simulink library "thc"  (R2021b)
settings: Solver=VariableStepAuto  StartTime=0.0  StopTime=10.0  RelTol=1e-3
undefined symbols (not defined in the file or in its folder): ATHC_APTCQA_X_C, ATHC_APTCQB_X_C, ATHC_dAy_X_C, ATHC_Qeq_X_kmh, ATHC_VbaseC_X_C, ATHC_VbaseC_Y_W, ATHC_VbaseD_X_C, ATHC_VbaseH_X_C, KTHC_ACMaxMinT_sec, KTHC_aDeice_K, KTHC_AGSDefLv_K, KTHC_AGSLv1_K, KTHC_AGSLv2_K, KTHC_AGSLv3_K, KTHC_AGSLv4_K, KTHC_AGSLv5_K, KTHC_AirIntUpdateT_sec, KTHC_APTCOneZoneMax_W, KTHC_APTCPeriod_cnt, KTHC_APTCPWMEN_flg, KTHC_APTCQMaxC_W, KTHC_APTCQminC_W, KTHC_APTCQminD_W, KTHC_APTCQminRe1_W, KTHC_APTCQminRe_W, KTHC_APTCQoffT_cnt, KTHC_APTCQonT_cnt, KTHC_APTCRiLeMaxDff_W, KTHC_APTCRiLeMinDff_W, KTHC_AutoWDTamb1_C, KTHC_AutoWDTamb2_C, KTHC_AutoWDTamb3_C, KTHC_BatCoolT_cnt, KTHC_BatInTempDef_C, KTHC_bDeice_K, KTHC_CompMaxDeice_rpm, KTHC_CompMinDeice_rpm, KTHC_CompSotxvOp_K, KTHC_CompSotxvOpLow_rpm, KTHC_CompSpdEXVUp1_rpm, KTHC_CompSpdEXVUp2_rpm, KTHC_CompSpdEXVUp3_rpm, KTHC_CompSpdEXVUp4_rpm, KTHC_CompSpdmax_rpm, KTHC_CompSpdmaxBC1_rpm, KTHC_CompSpdmaxBC_rpm, KTHC_CompSpdmid1_rpm, KTHC_CompSpdmid2_rpm, KTHC_CompSpdmid3_rpm, KTHC_CompSpdmid4_rpm, KTHC_CompSpdmid5_rpm, KTHC_CompSpdmid_rpm, KTHC_CompSpdmin_rpm, KTHC_DAPTCQ1_W, KTHC_DAPTCQ2_W, KTHC_DAPTCQ3_W, KTHC_DcChSetTemp_C, KTHC_DehumidityEN_flg, KTHC_DeiceCycTime_K, KTHC_DriveLevelWPTCBAH1_W ... (+403)
libraries: simulink x489
(part 2 of 18)

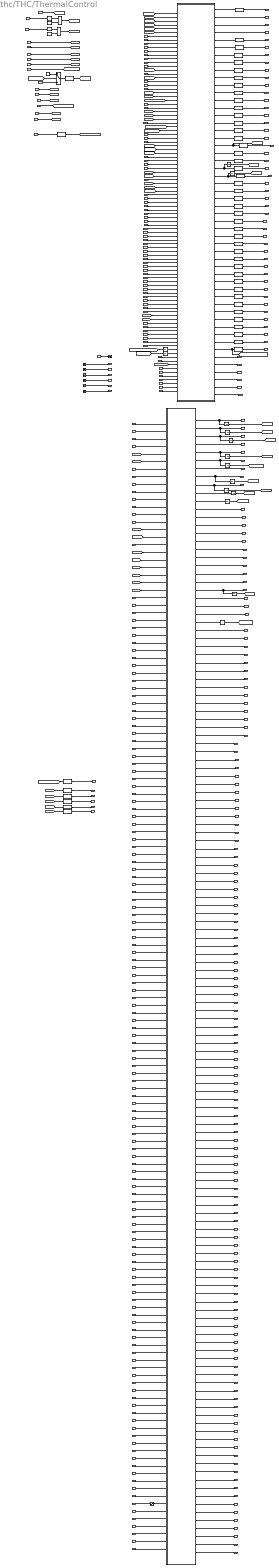
== system thc/THC/ThermalControl ==
  note: Ver Infomation
      | THCM Model V92A
      | ACHMI Model V33A
  VPMM_PwrSta_enum : Inport
  VPMM_SysPwrSta_enum : Inport  Port=2
  VTQD_ShiftGearPosn_enum : Inport  Port=3
  VSCP_AGSCloseSta_flg : Inport  Port=4
  VINP_VehSpeed_kph : Inport  Port=5
  VINP_HVBMTempMax_C : Inport  Port=6
  VINP_HVBMTempMin_C : Inport  Port=7
  VINP_OBCTemp_C : Inport  Port=8
  VINP_DCDCTemp_C : Inport  Port=9
  VINP_RrTMTemp_C : Inport  Port=10
  VINP_RrMCUTemp_C : Inport  Port=11
  VINP_FrTMTemp_C : Inport  Port=12
  VINP_FrMCUTemp_C : Inport  Port=13
  VINP_ChrgPlugSta_enum : Inport  Port=14
  VINP_FrLLCTemp_C : Inport  Port=15
  VINP_RrLLCTemp_C : Inport  Port=16
  VINP_HVBIsoImpedenceN_Mohm : Inport  Port=17
  VINP_HVBIsoImpedenceP_Mohm : Inport  Port=18
  VINP_HVBHVILErr_flg : Inport  Port=19
  VINP_HVBattSOC_pct : Inport  Port=20
  VINP_PTHighTact_C : Inport  Port=21
  VINP_COMP_StatorSpd_RPM : Inport  Port=22
  VINP_CompProEN_flg : Inport  Port=23
  VINP_PTLowP1_kPa : Inport  Port=24
  VINP_PTLowT1_C : Inport  Port=25
  VINP_PTLowP2_kPa : Inport  Port=26
  VINP_PTLowT2_C : Inport  Port=27
  VINP_PTHighP_kPa : Inport  Port=28
  VINP_Tamb_C : Inport  Port=29
  VINP_BatInTemp_C : Inport  Port=30
  VINP_BatOutTemp_C : Inport  Port=31
  VINP_MotorInTemp_C : Inport  Port=32
  VINP_MotorOutTemp_C : Inport  Port=33
  VINP_Tincar_C : Inport  Port=34
  VINP_SolarL_W : Inport  Port=35
  VINP_SolarR_W : Inport  Port=36
  VINP_Tevap_C : Inport  Port=37
  VINP_TFaceL_C : Inport  Port=38
  VINP_TFaceR_C : Inport  Port=39
  VINP_TFootL_C : Inport  Port=40
  VINP_TFootR_C : Inport  Port=41
  VINP_TFootRr_C : Inport  Port=42
  VINP_TFaceRr_C : Inport  Port=43
  VINP_EACProtectEnable_enum : Inport  Port=44
  Tamb_Err : Inport  Port=45
  SolarL_Err : Inport  Port=46
  SolarR_Err : Inport  Port=47
  Tevap_Err : Inport  Port=48
  T_Face_L_Err : Inport  Port=49
  T_Face_R_Err : Inport  Port=50
  T_Foot_L_Err : Inport  Port=51
  T_Foot_R_Err : Inport  Port=52
  T_Face_Rr_Err : Inport  Port=53
  T_Foot_Rr_Err : Inport  Port=54
  Tincar_Err : Inport  Port=55
  Bat_In_Temp_Err : Inport  Port=56
  Motor_In_Temp_Err : Inport  Port=57
  Motor_Out_Temp_Err : Inport  Port=58
  Fan_Err : Inport  Port=59
  AGS_Err : Inport  Port=60
  EWP3_Err : Inport  Port=61
  PT_High_P_Err : Inport  Port=62
  PT_High_Tact_Err : Inport  Port=63
  SOV1_Err : Inport  Port=64
  SOV2_Err : Inport  Port=65
  SOV3_Err : Inport  Port=66
  EXV1_Err : Inport  Port=67
  EXV2_Err : Inport  Port=68
  Comp_Err : Inport  Port=69
  Blower_Err : Inport  Port=70
  PT_Low_P1_Err : Inport  Port=71
  PT_Low_T1_Err : Inport  Port=72
  PT_Low_P2_Err : Inport  Port=73
  PT_Low_T2_Err : Inport  Port=74
  SOTXV_Err : Inport  Port=75
  VINP_FrntPTCRearLeActHeatPwr_W : Inport  Port=76
  VINP_FrntPTCLeActHeatPwr_W : Inport  Port=77
  VINP_FrntPTCRiActHeatPwr_W : Inport  Port=78
  VINP_ZFRTHCLEVentActYSta_enum : Inport  Port=79
  VINP_ZFRTHCCLEVentActYSta_enum : Inport  Port=80
  VINP_ZFRTHCREVentActYSta_enum : Inport  Port=81
  VINP_ZFRTHCCREVentActYSta_enum : Inport  Port=82
  VINP_FGSAirIntSta_enum : Inport  Port=83
  "VINP_EWP1BlockError_enum " : Inport  Port=84
  VINP_EWP1OverCurrError_enum : Inport  Port=85
  VINP_EWP2BlockError_enum : Inport  Port=86
  VINP_EWP2OverCurrError_enum : Inport  Port=87
  VINP_EWP3BlockError_enum : Inport  Port=88
  VINP_EWP3OverCurrError_enum : Inport  Port=89
  VINP_OFFACMODE_enum : Inport  Port=90
  VINP_FCPFrEvtBtnACMaxReq_flg : Inport  Port=91
  VINP_FCPFrEvtBtnACReq_flg : Inport  Port=92
  VINP_FCPFrEvtBtnAutoReq_flg : Inport  Port=93
  VINP_FCPFrEvtBtnSyncReq_flg : Inport  Port=94
  VINP_sigAirIntenZon1Req_enum : Inport  Port=95
  VINP_sigRecircReq_flg : Inport  Port=96
  VINP_sigFaceReq_flg : Inport  Port=97
  VINP_sigFootReq_flg : Inport  Port=98
  VINP_sigFrostReq_flg : Inport  Port=99
  VINP_sigSetTempZon1Req_C : Inport  Port=100
  VINP_CANMsgValidIVI2_flg : Inport  Port=101
  VINP_sigSetTempZon2Req_C : Inport  Port=102
  VINP_SmartEcoModeSW_flg : Inport  Port=103
  VINP_HMIACBtnCmd_flg : Inport  Port=104
  VINP_HMIACAutoBtnCmd_flg : Inport  Port=105
  VINP_HMIACRecycleBtnCmd_flg : Inport  Port=106
  VINP_HMIACFrDefogBtnCmd_flg : Inport  Port=107
  VINP_HMIZLSetTPCmd_flg : Inport  Port=108
  VINP_HMIZLSetTMCmd_flg : Inport  Port=109
  VINP_HMIZRSetTPCmd_flg : Inport  Port=110
  VINP_HMIZRSetTMCmd_flg : Inport  Port=111
  VINP_HMIACWindDirPCmd_flg : Inport  Port=112
  VINP_HMIACWindDirMCmd_flg : Inport  Port=113
  VINP_HMIACAirIntPCmd_flg : Inport  Port=114
  VINP_HMIACAirIntMCmd_flg : Inport  Port=115
  VINP_IVIAirIntZ3Cmd_enum : Inport  Port=116
  VINP_IVILBlowerModeSta_enum : Inport  Port=117
  VINP_IVIRBlowerModeSta_enum : Inport  Port=118
  VINP_IVILBlowerZSta_enum : Inport  Port=119
  VINP_IVICLBlowerZSta_enum : Inport  Port=120
  VINP_IVIRBlowerZSta_enum : Inport  Port=121
  VINP_IVICRBlowerZSta_enum : Inport  Port=122
  VINP_IVILBlowerYSta_enum : Inport  Port=123
  VINP_IVICLBlowerYSta_enum : Inport  Port=124
  VINP_IVIRBlowerYSta_enum : Inport  Port=125
  VINP_IVICRBlowerYSta_enum : Inport  Port=126
  VINP_IVIsigScreenReq_Sta : Inport  Port=127
  VINP_IVIFGSAirIntCmd_enum : Inport  Port=128
  VINP_IVIFGSChCmd_enum : Inport  Port=129
  VINP_IVIIONSWCmd_flg : Inport  Port=130
  VINP_IVIWPTCSWSta_flg : Inport  Port=131
  VINP_IVIZon1WindDirSWReqSta_flg : Inport  Port=132
  VINP_IVIQuickRefreshSta_flg : Inport  Port=133
  ECOSW : Inport  Port=134
  VINP_RemoteACTemp_C : Inport  Port=135
  VINP_RemoteAutoReq_flg : Inport  Port=136
  EEP_ACModeSet123 : Inport  Port=137
  EEP_FACESet : Inport  Port=138
  EEP_FOOTSet : Inport  Port=139
  EEP_FrostSet : Inport  Port=140
  EEP_FaceMSet : Inport  Port=141
  EEP_FootMSet : Inport  Port=142
  EEP_CCUSyncStsSet : Inport  Port=143
  EEP_sigRecircStSet : Inport  Port=144
  EEP_RecyAutoSet : Inport  Port=145
  EEP_AirIntenZone1MSet1 : Inport  Port=146
  EEP_fdefogSet : Inport  Port=147
  EEP_SettempZon1Set1 : Inport  Port=148
  EEP_sigSetTempZon2StM : Inport  Port=149
  EEP_AirIntenZone3MSet1 : Inport  Port=150
  EEP_FDCTHCREVentModeStaSet123 : Inport  Port=151
  EEP_FDCTHCLEVentModeStaSet123 : Inport  Port=152
  EEP_FDCTHCLEVentZStaSet1 : Inport  Port=153
  EEP_FDCTHCCLEVentZStaSet1 : Inport  Port=154
  EEP_FDCTHCREVentZStaSet1 : Inport  Port=155
  EEP_FDCTHCCREVentZStaSet1 : Inport  Port=156
  EEP_LVentENSet : Inport  Port=157
  EEP_FDCTHCLEVentYStaSet1 : Inport  Port=158
  EEP_CLVentENSet : Inport  Port=159
  EEP_FDCTHCCLEVentYStaSet1 : Inport  Port=160
  EEP_RVentENSet : Inport  Port=161
  EEP_FDCTHCREVentYStaSet1 : Inport  Port=162
  EEP_CRVentENSet : Inport  Port=163
  EEP_FDCTHCCREVentYStaSet1 : Inport  Port=164
  EEP_FDCFGSAirIntStaSet123 : Inport  Port=165
  EEP_FDCFGSChStaSet123 : Inport  Port=166
  EEP_IONSWStaSet : Inport  Port=167
  EEP_AirIntenZone1MSet2 : Inport  Port=168
  EEP_AirIntenZone1MSet3 : Inport  Port=169
  EEP_AirIntenZone1MSet4 : Inport  Port=170
  EEP_AirIntenZone1MSet5 : Inport  Port=171
  EEP_AirIntenZone1MSet7 : Inport  Port=172
  EEP_AirIntenZone3MSet2 : Inport  Port=173
  EEP_AirIntenZone3MSet3 : Inport  Port=174
  EEP_AirIntenZone3MSet4 : Inport  Port=175
  EEP_AirIntenZone3MSet5 : Inport  Port=176
  EEP_AirIntenZone3MSet7 : Inport  Port=177
  EEP_FDCFGSChStaSet457 : Inport  Port=178
  EEP_FDCFGSAirIntStaSet457 : Inport  Port=179
  EEP_FDCTHCLEVentModeStaSet457 : Inport  Port=180
  EEP_FDCTHCREVentModeStaSet457 : Inport  Port=181
  EEP_FDCTHCLEVentZStaSet2 : Inport  Port=182
  EEP_FDCTHCLEVentZStaSet3 : Inport  Port=183
  EEP_FDCTHCLEVentZStaSet4 : Inport  Port=184
  EEP_FDCTHCLEVentZStaSet5 : Inport  Port=185
  EEP_FDCTHCLEVentZStaSet7 : Inport  Port=186
  EEP_FDCTHCCLEVentZStaSet2 : Inport  Port=187
  EEP_FDCTHCCLEVentZStaSet3 : Inport  Port=188
  EEP_FDCTHCCLEVentZStaSet4 : Inport  Port=189
  EEP_FDCTHCCLEVentZStaSet5 : Inport  Port=190
  EEP_FDCTHCCLEVentZStaSet7 : Inport  Port=191
  EEP_FDCTHCREVentZStaSet2 : Inport  Port=192
  EEP_FDCTHCREVentZStaSet3 : Inport  Port=193
  EEP_FDCTHCREVentZStaSet4 : Inport  Port=194
  EEP_FDCTHCREVentZStaSet5 : Inport  Port=195
  EEP_FDCTHCREVentZStaSet7 : Inport  Port=196
  EEP_FDCTHCCREVentZStaSet2 : Inport  Port=197
  EEP_FDCTHCCREVentZStaSet3 : Inport  Port=198
  EEP_FDCTHCCREVentZStaSet4 : Inport  Port=199
  EEP_FDCTHCCREVentZStaSet5 : Inport  Port=200
  EEP_FDCTHCCREVentZStaSet7 : Inport  Port=201
  EEP_FDCTHCLEVentYStaSet2 : Inport  Port=202
  EEP_FDCTHCLEVentYStaSet3 : Inport  Port=203
  EEP_FDCTHCLEVentYStaSet4 : Inport  Port=204
  EEP_FDCTHCLEVentYStaSet5 : Inport  Port=205
  EEP_FDCTHCLEVentYStaSet7 : Inport  Port=206
  EEP_FDCTHCCLEVentYStaSet2 : Inport  Port=207
  EEP_FDCTHCCLEVentYStaSet3 : Inport  Port=208
  EEP_FDCTHCCLEVentYStaSet4 : Inport  Port=209
  EEP_FDCTHCCLEVentYStaSet5 : Inport  Port=210
  EEP_FDCTHCCLEVentYStaSet7 : Inport  Port=211
  EEP_FDCTHCREVentYStaSet2 : Inport  Port=212
  EEP_FDCTHCREVentYStaSet3 : Inport  Port=213
  EEP_FDCTHCREVentYStaSet4 : Inport  Port=214
  EEP_FDCTHCREVentYStaSet5 : Inport  Port=215
  EEP_FDCTHCREVentYStaSet7 : Inport  Port=216
  EEP_FDCTHCCREVentYStaSet2 : Inport  Port=217
  EEP_FDCTHCCREVentYStaSet3 : Inport  Port=218
  EEP_FDCTHCCREVentYStaSet4 : Inport  Port=219
  EEP_FDCTHCCREVentYStaSet5 : Inport  Port=220
  EEP_FDCTHCCREVentYStaSet7 : Inport  Port=221
  EEP_ACModeSet457 : Inport  Port=222
  EEP_SettempZon1Set2 : Inport  Port=223
  EEP_SettempZon1Set3 : Inport  Port=224
  EEP_SettempZon1Set4 : Inport  Port=225
  EEP_SettempZon1Set5 : Inport  Port=226
  EEP_SettempZon1Set7 : Inport  Port=227
  VBCM_UserNow_enum : Inport  Port=228
  VINP_UpdateReq_enum : Inport  Port=229
  APTCFailDTC : Inport  Port=230
  AC : Subsystem
  Abs : Abs
  Abs1 : Abs
  Constant : Constant
  Constant1 : Constant
  Constant2 : Constant  Value=2
  Data Type Conversion{,1..47,50} (49 alike) : DataTypeConversion
  Data Type Conversion48 : DataTypeConversion  OutDataTypeStr=uint8
  Data Type Conversion49 : DataTypeConversion  OutDataTypeStr=uint16
  Ground{,1..5} (6 alike) : Ground
  Max : MinMax  Function=max  Inputs=2
  Max1 : MinMax  Function=max  Inputs=2
  Saturation : Saturate  UpperLimit=30  LowerLimit=0
  Switch : Switch  Criteria=u2 > Threshold
  THCM_Conctrl : Subsystem
  Terminator : Terminator
  Unit Delay{,1..14} (15 alike) : UnitDelay  SampleTime=-1  HasFrameUpgradeWarning=on
  VTHC_FDCompCmd_rpm : Outport
  VTHC_FDSOV1Cmd_flg : Outport  Port=2
  VTHC_FDSOV2Cmd_flg : Outport  Port=3
  VTHC_FDSOV3Cmd_flg : Outport  Port=4
  VTHC_FDEXV1Cmd_step : Outport  Port=5
  VTHC_FDEXV2Cmd_step : Outport  Port=6
  VTHC_FDSOTXVCmd_flg : Outport  Port=7
  VTHC_FDFWVCmd_flg : Outport  Port=8
  VTHC_FDTWVCmd_pct : Outport  Port=9
  VTHC_FDFrWPTCHeatPwrCmd_W : Outport  Port=10
  VTHC_CoolgFanActDuty_pct : Outport  Port=11
  VTHC_FDAGSCmd_enum : Outport  Port=12
  VTHC_FDEWP1Cmd_enum : Outport  Port=13
  VTHC_FDEWP2Cmd_enum : Outport  Port=14
  VTHC_FDEWP3Cmd_enum : Outport  Port=15
  VTHC_FDFrLeAPTCHeatPwrCmd_W : Outport  Port=16
  VTHC_FDFrRiAPTCHeatPwrCmd_W : Outport  Port=17
  VTHC_FDRrAPTCHeatPwrCmd_W : Outport  Port=18
  VTHC_FDBlowerCmd_pct : Outport  Port=19
  VTHC_BatteryMode_enum : Outport  Port=20
  VTHC_EDriveMode_enum : Outport  Port=21
  VTHC_CabinMode_enum : Outport  Port=22
  VTHC_CCUACLampSts_flg : Outport  Port=23
  VTHC_CCUAutoLampSts_flg : Outport  Port=24
  VTHC_CCUACMaxLampSts_flg : Outport  Port=25
  VTHC_CCUSyncLampSts_flg : Outport  Port=26
  VTHC_sigAirIntenZon1St_enum : Outport  Port=27
  VTHC_sigWindDirZon1St_enum : Outport  Port=28
  VTHC_sigRecircSt_flg : Outport  Port=29
  VTHC_sigSetTempZon1St_C : Outport  Port=30
  VTHC_sigSetTempZon2St_C : Outport  Port=31
  VTHC_sigClntTHvBattOut_C : Outport  Port=32
  VTHC_sigCbnSolarLeft_W : Outport  Port=33
  VTHC_sigClntTHvBattIn_C : Outport  Port=34
  VTHC_sigCbnSolarRight_W : Outport  Port=35
  VTHC_sigAmbAirT_C : Outport  Port=36
  VTHC_sigCbnAirT_C : Outport  Port=37
  VTHC_ACSubMode_enum : Outport  Port=38
  VTHC_FDRecyAutoCmd_enum : Outport  Port=39
  VTHC_CompP_K : Outport  Port=40
  VTHC_CompI_K : Outport  Port=41
  VTHC_CompU_K : Outport  Port=42
  VTHC_CompDeltaU_K : Outport  Port=43
  VTHC_Compe_K : Outport  Port=44
  VTHC_Blowere_K : Outport  Port=45
  VTHC_BlowerP_K : Outport  Port=46
  VTHC_BlowerU_K : Outport  Port=47
  VTHC_Vbase_pct : Outport  Port=48
  VTHC_BlowerI_K : Outport  Port=49
  VTHC_EXV2P_K : Outport  Port=50
  VTHC_EXV2I_K : Outport  Port=51
  VTHC_EXV2U_K : Outport  Port=52
  VTHC_EXV2e_K : Outport  Port=53
  VTHC_APTCP_K : Outport  Port=54
  VTHC_APTCI_K : Outport  Port=55
  VTHC_APTCU_K : Outport  Port=56
  VTHC_APTCe_K : Outport  Port=57
  VTHC_EXV1P_K : Outport  Port=58
  VTHC_EXV1I_K : Outport  Port=59
  VTHC_EXV1U_K : Outport  Port=60
  VTHC_EXV1e_K : Outport  Port=61
  VTHC_ACModeMem_enum : Outport  Port=62
  VTHC_Face_flg : Outport  Port=63
  VTHC_Foot_flg : Outport  Port=64
  VTHC_Frost_flg : Outport  Port=65
  VTHC_FaceM_flg : Outport  Port=66
  VTHC_FootM_flg : Outport  Port=67
  VTHC_CCUSyncSts_flg : Outport  Port=68
  VTHC_RecAutoFlg_flg : Outport  Port=69
  VTHC_AirIntenZone1M_enum : Outport  Port=70
  VTHC_fdefog_flg : Outport  Port=71
  VTHC_sigSetTempZon2StM_C : Outport  Port=72
  VTHC_sigDfrstSt_flg : Outport  Port=73
  VTHC_FDCTHCAirIntZ3Sta_enum : Outport  Port=74
  VTHC_FDCTHCLEVentModeSta_enum : Outport  Port=75
  VTHC_FDCTHCREVentModeSta_enum : Outport  Port=76
  VTHC_FDCTHCLEVentZSta_enum : Outport  Port=77
  VTHC_FDCTHCCLEVentZSta_enum : Outport  Port=78
  VTHC_FDCTHCREVentZSta_enum : Outport  Port=79
  VTHC_FDCTHCCREVentZSta_enum : Outport  Port=80
  VTHC_FDCTHCLEVentYSta_enum : Outport  Port=81
  VTHC_FDCTHCLVentENSta_flg : Outport  Port=82
  VTHC_FDCTHCCLEVentYSta_enum : Outport  Port=83
  VTHC_FDCTHCCLVentENSta_flg : Outport  Port=84
  VTHC_FDCTHCREVentYSta_enum : Outport  Port=85
  VTHC_FDCTHCRVentENSta_flg : Outport  Port=86
  VTHC_FDCTHCCREVentYSta_enum : Outport  Port=87
  VTHC_FDCTHCCRVentENSta_flg : Outport  Port=88
  VTHC_FDCTHCMAPTCForceOFFSta_flg : Outport  Port=89
  VTHC_Z1TUP_flg : Outport  Port=90
  VTHC_Z1TDN_flg : Outport  Port=91
  VTHC_Z2TUP_flg : Outport  Port=92
  VTHC_Z2TDN_flg : Outport  Port=93
  VTHC_FDCFGSAirIntSta_enum : Outport  Port=94
  VTHC_FDCFGSChSta_enum : Outport  Port=95
  VTHC_FDCFGSAirIntCmd_enum : Outport  Port=96
  VTHC_FDCFGSFuncSta_enum : Outport  Port=97
  VTHC_FDCFGSChCmd_enum : Outport  Port=98
  VTHC_FDCFGSIONSWSta_flg : Outport  Port=99
  VTHC_FDCFGSIONCmd_flg : Outport  Port=100
  VTHC_FDCTHCMPreWPTCHeatSta_enum : Outport  Port=101
  VTHC_EWPBUflag1_flg : Outport  Port=102
  VTHC_EWPBUflag2_flg : Outport  Port=103
  VTHC_EWPBUflag3_flg : Outport  Port=104
  VTHC_FaceMSet_enum : Outport  Port=105
  VTHC_FootMSet_enum : Outport  Port=106
  VTHC_fdefogSet_enum : Outport  Port=107
  VTHC_CCUSyncStsSet_enum : Outport  Port=108
  VTHC_sigRecircStSet_enum : Outport  Port=109
  VTHC_RecyAutoSet_enum : Outport  Port=110
  VTHC_AirIntenZone1MSet1_enum : Outport  Port=111
  VTHC_AirIntenZone1MSet2_enum : Outport  Port=112
  VTHC_AirIntenZone1MSet3_enum : Outport  Port=113
  VTHC_AirIntenZone1MSet4_enum : Outport  Port=114
  VTHC_AirIntenZone1MSet5_enum : Outport  Port=115
  VTHC_AirIntenZone1MSet7_enum : Outport  Port=116
  VTHC_AirIntenZone3MSet1_enum : Outport  Port=117
  VTHC_AirIntenZone3MSet2_enum : Outport  Port=118
  VTHC_AirIntenZone3MSet3_enum : Outport  Port=119
  VTHC_AirIntenZone3MSet4_enum : Outport  Port=120
  VTHC_AirIntenZone3MSet5_enum : Outport  Port=121
  VTHC_AirIntenZone3MSet7_enum : Outport  Port=122
  VTHC_IONSWStaSet_enum : Outport  Port=123
  VTHC_FDCFGSChStaSet123_enum : Outport  Port=124
  VTHC_FDCFGSChStaSet457_enum : Outport  Port=125
  VTHC_FDCFGSAirIntStaSet123_enum : Outport  Port=126
  VTHC_FDCFGSAirIntStaSet457_enum : Outport  Port=127
  VTHC_LVentENSet_enum : Outport  Port=128
  VTHC_CLVentENSet_enum : Outport  Port=129
  VTHC_RVentENSet_enum : Outport  Port=130
  VTHC_CRVentENSet_enum : Outport  Port=131
  VTHC_LEVentModeStaSet123_enum : Outport  Port=132
  VTHC_LEVentModeStaSet457_enum : Outport  Port=133
  VTHC_REVentModeStaSet123_enum : Outport  Port=134
  VTHC_REVentModeStaSet457_enum : Outport  Port=135
  VTHC_FDCTHCLEVentZStaSet1_enum : Outport  Port=136
  VTHC_FDCTHCLEVentZStaSet2_enum : Outport  Port=137
  VTHC_FDCTHCLEVentZStaSet3_enum : Outport  Port=138
  VTHC_FDCTHCLEVentZStaSet4_enum : Outport  Port=139
  VTHC_FDCTHCLEVentZStaSet5_enum : Outport  Port=140
  VTHC_FDCTHCLEVentZStaSet7_enum : Outport  Port=141
  VTHC_FDCTHCCLEVentZStaSet1_enum : Outport  Port=142
  VTHC_FDCTHCCLEVentZStaSet2_enum : Outport  Port=143
  VTHC_FDCTHCCLEVentZStaSet3_enum : Outport  Port=144
  VTHC_FDCTHCCLEVentZStaSet4_enum : Outport  Port=145
  VTHC_FDCTHCCLEVentZStaSet5_enum : Outport  Port=146
  VTHC_FDCTHCCLEVentZStaSet7_enum : Outport  Port=147
  VTHC_FDCTHCREVentZStaSet1_enum : Outport  Port=148
  VTHC_FDCTHCREVentZStaSet2_enum : Outport  Port=149
  VTHC_FDCTHCREVentZStaSet3_enum : Outport  Port=150
  VTHC_FDCTHCREVentZStaSet4_enum : Outport  Port=151
  VTHC_FDCTHCREVentZStaSet5_enum : Outport  Port=152
  VTHC_FDCTHCREVentZStaSet7_enum : Outport  Port=153
  VTHC_FDCTHCCREVentZStaSet1_enum : Outport  Port=154
  VTHC_FDCTHCCREVentZStaSet2_enum : Outport  Port=155
  VTHC_FDCTHCCREVentZStaSet3_enum : Outport  Port=156
  VTHC_FDCTHCCREVentZStaSet4_enum : Outport  Port=157
  VTHC_FDCTHCCREVentZStaSet5_enum : Outport  Port=158
  VTHC_FDCTHCCREVentZStaSet7_enum : Outport  Port=159
  VTHC_FDCTHCLEVentYStaSet1_enum : Outport  Port=160
  VTHC_FDCTHCLEVentYStaSet2_enum : Outport  Port=161
  VTHC_FDCTHCLEVentYStaSet3_enum : Outport  Port=162
  VTHC_FDCTHCLEVentYStaSet4_enum : Outport  Port=163
  VTHC_FDCTHCLEVentYStaSet5_enum : Outport  Port=164
  VTHC_FDCTHCLEVentYStaSet7_enum : Outport  Port=165
  VTHC_FDCTHCCLEVentYStaSet1_enum : Outport  Port=166
  VTHC_FDCTHCCLEVentYStaSet2_enum : Outport  Port=167
  VTHC_FDCTHCCLEVentYStaSet3_enum : Outport  Port=168
  VTHC_FDCTHCCLEVentYStaSet4_enum : Outport  Port=169
  VTHC_FDCTHCCLEVentYStaSet5_enum : Outport  Port=170
  VTHC_FDCTHCCLEVentYStaSet7_enum : Outport  Port=171
  VTHC_FDCTHCREVentYStaSet1_enum : Outport  Port=172
  VTHC_FDCTHCREVentYStaSet2_enum : Outport  Port=173
  VTHC_FDCTHCREVentYStaSet3_enum : Outport  Port=174
  VTHC_FDCTHCREVentYStaSet4_enum : Outport  Port=175
  VTHC_FDCTHCREVentYStaSet5_enum : Outport  Port=176
  VTHC_FDCTHCREVentYStaSet7_enum : Outport  Port=177
  VTHC_FDCTHCCREVentYStaSet1_enum : Outport  Port=178
  VTHC_FDCTHCCREVentYStaSet2_enum : Outport  Port=179
  VTHC_FDCTHCCREVentYStaSet3_enum : Outport  Port=180
  VTHC_FDCTHCCREVentYStaSet4_enum : Outport  Port=181
  VTHC_FDCTHCCREVentYStaSet5_enum : Outport  Port=182
  VTHC_FDCTHCCREVentYStaSet7_enum : Outport  Port=183
  VTHC_SettempZon1Set1_enum : Outport  Port=184
  VTHC_SettempZon1Set2_enum : Outport  Port=185
  VTHC_SettempZon1Set3_enum : Outport  Port=186
  VTHC_SettempZon1Set4_enum : Outport  Port=187
  VTHC_SettempZon1Set5_enum : Outport  Port=188
  VTHC_SettempZon1Set7_enum : Outport  Port=189
  VTHC_ACModeSet123_enum : Outport  Port=190
  VTHC_ACModeSet457_enum : Outport  Port=191
  VTHC_FACESet_enum : Outport  Port=192
  VTHC_FOOTSet_enum : Outport  Port=193
  VTHC_FrostSet_enum : Outport  Port=194
  VTHC_LVentEN_flg : Outport  Port=195
  VTHC_CLVentEN_flg : Outport  Port=196
  VTHC_RVentEN_flg : Outport  Port=197
  VTHC_CRVentEN_flg : Outport  Port=198
  VTHC_FDCFGSLearnCmd_enum : Outport  Port=199
  VTHC_FDCFGSFuncSta_flg : Outport  Port=200
  VTHC_THSysErrlampReq_flg : Outport  Port=201
  VTHC_sigCbnPTCPwrAct_W : Outport  Port=202
  wires:
  THCM_Conctrl/51(VTHC_THSysErrlampReq_flg) -> VTHC_THSysErrlampReq_flg/1  "VTHC_THSysErrlampReq_flg"
  VPMM_SysPwrSta_enum/1 -> THCM_Conctrl/101(VPMM_SysPwrSta_enum)
  Ground5/1 -> VTHC_FDCFGSFuncSta_flg/1  "VTHC_FDCFGSFuncSta_flg"
  Saturation/1 -> AC/144(EEP_SettempZon1Set1)
  Ground4/1 -> VTHC_FDCFGSLearnCmd_enum/1  "VTHC_FDCFGSLearnCmd_enum"
  Ground2/1 -> VTHC_RVentEN_flg/1  "VTHC_RVentEN_flg"
  Ground3/1 -> VTHC_CRVentEN_flg/1  "VTHC_CRVentEN_flg"
  Ground1/1 -> VTHC_CLVentEN_flg/1  "VTHC_CLVentEN_flg"
  Ground/1 -> VTHC_LVentEN_flg/1  "VTHC_LVentEN_flg"
  AC/56(FrostSet) -> VTHC_FrostSet_enum/1  "VTHC_FrostSet_enum"
  AC/55(FOOTSet) -> VTHC_FOOTSet_enum/1  "VTHC_FOOTSet_enum"
  AC/54(FACESet) -> VTHC_FACESet_enum/1  "VTHC_FACESet_enum"
  AC/53(ACModeSet457) -> VTHC_ACModeSet457_enum/1  "VTHC_ACModeSet457_enum"
  AC/52(ACModeSet123) -> VTHC_ACModeSet123_enum/1  "VTHC_ACModeSet123_enum"
  AC/51(VTHC_FDCFGSIONCmd_flg) -> VTHC_FDCFGSIONCmd_flg/1  "VTHC_FDCFGSIONCmd_flg"
  AC/50(VTHC_FDCFGSIONSWSta_flg) -> VTHC_FDCFGSIONSWSta_flg/1  "VTHC_FDCFGSIONSWSta_flg"
  AC/49(VTHC_FDCFGSChCmd_enum) -> VTHC_FDCFGSChCmd_enum/1  "VTHC_FDCFGSChCmd_enum"
  AC/48(VTHC_FDCFGSFuncSta_enum) -> VTHC_FDCFGSFuncSta_enum/1  "VTHC_FDCFGSFuncSta_enum"
  AC/47(VTHC_FDCFGSAirIntCmd_enum) -> VTHC_FDCFGSAirIntCmd_enum/1  "VTHC_FDCFGSAirIntCmd_enum"
  AC/46(VTHC_FDCFGSChSta_enum) -> VTHC_FDCFGSChSta_enum/1  "VTHC_FDCFGSChSta_enum"
  AC/45(VTHC_FDCFGSAirIntSta_enum) -> VTHC_FDCFGSAirIntSta_enum/1  "VTHC_FDCFGSAirIntSta_enum"
  AC/44(VTHC_Z2TDN_flg) -> VTHC_Z2TDN_flg/1  "VTHC_Z2TDN_flg"
  AC/43(VTHC_Z2TUP_flg) -> VTHC_Z2TUP_flg/1  "VTHC_Z2TUP_flg"
  AC/42(VTHC_Z1TDN_flg) -> VTHC_Z1TDN_flg/1  "VTHC_Z1TDN_flg"
  AC/41(VTHC_Z1TUP_flg) -> VTHC_Z1TUP_flg/1  "VTHC_Z1TUP_flg"
  EEP_SettempZon1Set7/1 -> AC/149(EEP_SettempZon1Set7)
  EEP_SettempZon1Set5/1 -> AC/148(EEP_SettempZon1Set5)
  EEP_SettempZon1Set4/1 -> AC/147(EEP_SettempZon1Set4)
  EEP_SettempZon1Set3/1 -> AC/146(EEP_SettempZon1Set3)
  EEP_SettempZon1Set2/1 -> AC/145(EEP_SettempZon1Set2)
  EEP_SettempZon1Set1/1 -> Saturation/1
  EEP_FDCTHCCREVentYStaSet7/1 -> AC/143(EEP_FDCTHCCREVentYStaSet7)
  EEP_FDCTHCCREVentYStaSet5/1 -> AC/142(EEP_FDCTHCCREVentYStaSet5)
  EEP_FDCTHCCREVentYStaSet4/1 -> AC/141(EEP_FDCTHCCREVentYStaSet4)
  EEP_FDCTHCCREVentYStaSet3/1 -> AC/140(EEP_FDCTHCCREVentYStaSet3)
  EEP_FDCTHCCREVentYStaSet2/1 -> AC/139(EEP_FDCTHCCREVentYStaSet2)
  EEP_FDCTHCCREVentYStaSet1/1 -> AC/138(EEP_FDCTHCCREVentYStaSet1)
  EEP_FDCTHCREVentYStaSet7/1 -> AC/137(EEP_FDCTHCREventYStaSet7)
  EEP_FDCTHCREVentYStaSet5/1 -> AC/136(EEP_FDCTHCREventYStaSet5)
  EEP_FDCTHCREVentYStaSet4/1 -> AC/135(EEP_FDCTHCREventYStaSet4)
  EEP_FDCTHCREVentYStaSet3/1 -> AC/134(EEP_FDCTHCREventYStaSet3)
  EEP_FDCTHCREVentYStaSet2/1 -> AC/133(EEP_FDCTHCREventYStaSet2)
  EEP_FDCTHCREVentYStaSet1/1 -> AC/132(EEP_FDCTHCREventYStaSet1)
  EEP_FDCTHCCLEVentYStaSet7/1 -> AC/131(EEP_FDCTHCCLEVentYStaSet7)
  EEP_FDCTHCCLEVentYStaSet5/1 -> AC/130(EEP_FDCTHCCLEVentYStaSet5)
  EEP_FDCTHCCLEVentYStaSet4/1 -> AC/129(EEP_FDCTHCCLEVentYStaSet4)
  EEP_FDCTHCCLEVentYStaSet3/1 -> AC/128(EEP_FDCTHCCLEVentYStaSet3)
  EEP_FDCTHCCLEVentYStaSet2/1 -> AC/127(EEP_FDCTHCCLEVentYStaSet2)
  EEP_FDCTHCCLEVentYStaSet1/1 -> AC/126(EEP_FDCTHCCLEVentYStaSet1)
  EEP_FDCTHCLEVentYStaSet7/1 -> AC/125(EEP_FDCTHCLEventYStaSet7)
  EEP_FDCTHCLEVentYStaSet5/1 -> AC/124(EEP_FDCTHCLEventYStaSet5)
  EEP_FDCTHCLEVentYStaSet4/1 -> AC/123(EEP_FDCTHCLEventYStaSet4)
  EEP_FDCTHCLEVentYStaSet3/1 -> AC/122(EEP_FDCTHCLEventYStaSet3)
  EEP_FDCTHCLEVentYStaSet2/1 -> AC/121(EEP_FDCTHCLEventYStaSet2)
  EEP_FDCTHCCREVentZStaSet7/1 -> AC/119(EEP_FDCTHCCREVentZStaSet7)
  EEP_FDCTHCLEVentYStaSet1/1 -> AC/120(EEP_FDCTHCLEventYStaSet1)
  EEP_FDCTHCCREVentZStaSet5/1 -> AC/118(EEP_FDCTHCCREVentZStaSet5)
  EEP_FDCTHCCREVentZStaSet4/1 -> AC/117(EEP_FDCTHCCREVentZStaSet4)
  EEP_FDCTHCCREVentZStaSet3/1 -> AC/116(EEP_FDCTHCCREVentZStaSet3)
  EEP_FDCTHCCREVentZStaSet2/1 -> AC/115(EEP_FDCTHCCREVentZStaSet2)
  EEP_FDCTHCCREVentZStaSet1/1 -> AC/114(EEP_FDCTHCCREVentZStaSet1)
  EEP_FDCTHCREVentZStaSet7/1 -> AC/113(EEP_FDCTHCREventZStaSet7)
  EEP_FDCTHCREVentZStaSet5/1 -> AC/112(EEP_FDCTHCREventZStaSet5)
  EEP_FDCTHCREVentZStaSet4/1 -> AC/111(EEP_FDCTHCREventZStaSet4)
  EEP_FDCTHCREVentZStaSet3/1 -> AC/110(EEP_FDCTHCREventZStaSet3)
  EEP_FDCTHCREVentZStaSet2/1 -> AC/109(EEP_FDCTHCREventZStaSet2)
  EEP_FDCTHCREVentZStaSet1/1 -> AC/108(EEP_FDCTHCREventZStaSet1)
  EEP_FDCTHCCLEVentZStaSet7/1 -> AC/107(EEP_FDCTHCCLEVentZStaSet7)
  EEP_FDCTHCCLEVentZStaSet5/1 -> AC/106(EEP_FDCTHCCLEVentZStaSet5)
  EEP_FDCTHCCLEVentZStaSet4/1 -> AC/105(EEP_FDCTHCCLEVentZStaSet4)
  EEP_FDCTHCCLEVentZStaSet3/1 -> AC/104(EEP_FDCTHCCLEVentZStaSet3)
  EEP_FDCTHCCLEVentZStaSet2/1 -> AC/103(EEP_FDCTHCCLEVentZStaSet2)
  EEP_FDCTHCCLEVentZStaSet1/1 -> AC/102(EEP_FDCTHCCLEVentZStaSet1)
  EEP_FDCTHCLEVentZStaSet7/1 -> AC/101(EEP_FDCTHCLEventZStaSet7)
  EEP_FDCTHCLEVentZStaSet5/1 -> AC/100(EEP_FDCTHCLEventZStaSet5)
  EEP_FDCTHCLEVentZStaSet4/1 -> AC/99(EEP_FDCTHCLEventZStaSet4)
  EEP_FDCTHCLEVentZStaSet3/1 -> AC/98(EEP_FDCTHCLEventZStaSet3)
  EEP_FDCTHCLEVentZStaSet2/1 -> AC/97(EEP_FDCTHCLEventZStaSet2)
  EEP_FDCTHCLEVentZStaSet1/1 -> AC/96(EEP_FDCTHCLEventZStaSet1)
  EEP_FDCTHCREVentModeStaSet457/1 -> AC/95(EEP_FDCTHCREventModeStaSet457)
  EEP_FDCTHCREVentModeStaSet123/1 -> AC/94(EEP_FDCTHCREventModeStaSet123)
  EEP_FDCTHCLEVentModeStaSet457/1 -> AC/93(EEP_FDCTHCLEventModeStaSet457)
  EEP_FDCTHCLEVentModeStaSet123/1 -> AC/92(EEP_FDCTHCLEventModeStaSet123)
  EEP_CRVentENSet/1 -> AC/91(EEP_CRVentENSet)
  EEP_RVentENSet/1 -> AC/90(EEP_RVentENSet)
  EEP_CLVentENSet/1 -> AC/89(EEP_CLVentENSet)
  EEP_LVentENSet/1 -> AC/88(EEP_LVentENSet)
  EEP_FDCFGSAirIntStaSet457/1 -> AC/87(EEP_FDCFGSAirIntStaSet457)
  EEP_FDCFGSAirIntStaSet123/1 -> AC/86(EEP_FDCFGSAirIntStaSet123)
  EEP_FDCFGSChStaSet457/1 -> AC/85(EEP_FDCFGSChStaSet457)
  EEP_FDCFGSChStaSet123/1 -> AC/84(EEP_FDCFGSChStaSet123)
  EEP_IONSWStaSet/1 -> AC/83(EEP_IONSWStaSet)
  EEP_AirIntenZone3MSet7/1 -> AC/82(EEP_AirIntenZone3MSet7)
  EEP_AirIntenZone3MSet5/1 -> AC/81(EEP_AirIntenZone3MSet5)
  EEP_AirIntenZone3MSet4/1 -> AC/80(EEP_AirIntenZone3MSet4)
  EEP_AirIntenZone3MSet3/1 -> AC/79(EEP_AirIntenZone3MSet3)
  EEP_AirIntenZone3MSet2/1 -> AC/78(EEP_AirIntenZone3MSet2)
  EEP_AirIntenZone3MSet1/1 -> AC/77(EEP_AirIntenZone3MSet1)
  EEP_AirIntenZone1MSet7/1 -> AC/76(EEP_AirIntenZone1MSet7)
  EEP_AirIntenZone1MSet5/1 -> AC/75(EEP_AirIntenZone1MSet5)
  EEP_AirIntenZone1MSet4/1 -> AC/74(EEP_AirIntenZone1MSet4)
  EEP_AirIntenZone1MSet3/1 -> AC/73(EEP_AirIntenZone1MSet3)
  EEP_AirIntenZone1MSet1/1 -> AC/71(EEP_AirIntenZone1MSet1)
  EEP_AirIntenZone1MSet2/1 -> AC/72(EEP_AirIntenZone1MSet2)
  EEP_RecyAutoSet/1 -> AC/70(EEP_RecyAutoSet)
  EEP_sigRecircStSet/1 -> AC/69(EEP_sigRecircStSet)
  EEP_CCUSyncStsSet/1 -> AC/68(EEP_CCUSyncStsSet)
  EEP_fdefogSet/1 -> AC/67(EEP_fdefogSet)
  EEP_FootMSet/1 -> AC/66(EEP_FootMSet)
  EEP_FaceMSet/1 -> AC/65(EEP_FaceMSet)
  EEP_FrostSet/1 -> AC/64(EEP_FrostSet)
  EEP_FOOTSet/1 -> AC/63(EEP_FOOTSet)
  EEP_FACESet/1 -> AC/62(EEP_FACESet)
  EEP_ACModeSet457/1 -> AC/61(EEP_ACModeSet457)
  EEP_ACModeSet123/1 -> AC/60(EEP_ACModeSet123)
  VINP_UpdateReq_enum/1 -> AC/59(VINP_UpdateReq_enum)
  VBCM_UserNow_enum/1 -> AC/58(VBCM_UserNow_enum)
  VINP_IVIZon1WindDirSWReqSta_flg/1 -> AC/57(VINP_IVIZon1WindDirSWReqSta_flg)
  VINP_FGSAirIntSta_enum/1 -> AC/56(VINP_FGSAirIntSta_enum)
  VINP_IVIIONSWCmd_flg/1 -> AC/55(VINP_IVIIONSWCmd_flg)
  VINP_IVIFGSChCmd_enum/1 -> AC/54(VINP_IVIFGSChCmd_enum)
  VINP_IVIFGSAirIntCmd_enum/1 -> AC/53(VINP_IVIFGSAirIntCmd_enum)
  VINP_IVIsigScreenReq_Sta/1 -> AC/52(VINP_IVIsigScreenReq_Sta)
  VINP_ZFRTHCCREVentActYSta_enum/1 -> AC/51(VINP_ZFRTHCCREVentActYSta_enum)
  VINP_ZFRTHCREVentActYSta_enum/1 -> AC/50(VINP_ZFRTHCREventActYSta_enum)
  VINP_ZFRTHCCLEVentActYSta_enum/1 -> AC/49(VINP_ZFRTHCCLEVentActYSta_enum)
  VINP_IVICRBlowerYSta_enum/1 -> AC/47(VINP_IVICRBlowerYSta_enum)
  VINP_ZFRTHCLEVentActYSta_enum/1 -> AC/48(VINP_ZFRTHCLEventActYSta_enum)
  VINP_IVIRBlowerYSta_enum/1 -> AC/46(VINP_IVIRBlowerYSta_enum)
  VINP_IVICLBlowerYSta_enum/1 -> AC/45(VINP_IVICLBlowerYSta_enum)
  VINP_IVILBlowerYSta_enum/1 -> AC/44(VINP_IVILBlowerYSta_enum)
  VINP_IVICRBlowerZSta_enum/1 -> AC/43(VINP_IVICRBlowerZSta_enum)
  VINP_IVIRBlowerZSta_enum/1 -> AC/42(VINP_IVIRBlowerZSta_enum)
  VINP_IVICLBlowerZSta_enum/1 -> AC/41(VINP_IVICLBlowerZSta_enum)
  VINP_IVILBlowerZSta_enum/1 -> AC/40(VINP_IVILBlowerZSta_enum)
  VINP_IVIRBlowerModeSta_enum/1 -> AC/39(VINP_IVIRBlowerModeSta_enum)
  VINP_IVILBlowerModeSta_enum/1 -> AC/38(VINP_IVILBlowerModeSta_enum)
  VINP_IVIAirIntZ3Cmd_enum/1 -> AC/37(VINP_IVIAirIntZ3Cmd_enum)
  VINP_HMIACAirIntMCmd_flg/1 -> AC/36(VINP_HMIACAirIntMCmd_flg)
  VINP_HMIACAirIntPCmd_flg/1 -> AC/35(VINP_HMIACAirIntPCmd_flg)
  VINP_HMIACWindDirMCmd_flg/1 -> AC/34(VINP_HMIACWindDirMCmd_flg)
  VINP_HMIACWindDirPCmd_flg/1 -> AC/33(VINP_HMIACWindDirPCmd_flg)
  VINP_HMIZRSetTMCmd_flg/1 -> AC/32(VINP_HMIZRSetTMCmd_flg)
  VINP_HMIZRSetTPCmd_flg/1 -> AC/31(VINP_HMIZRSetTPCmd_flg)
  VINP_HMIZLSetTMCmd_flg/1 -> AC/30(VINP_HMIZLSetTMCmd_flg)
  VINP_HMIZLSetTPCmd_flg/1 -> AC/29(VINP_HMIZLSetTPCmd_flg)
  VINP_HMIACFrDefogBtnCmd_flg/1 -> AC/28(VINP_HMIACFrDefogBtnCmd_flg)
  VINP_HMIACRecycleBtnCmd_flg/1 -> AC/27(VINP_HMIACRecycleBtnCmd_flg)
  VINP_HMIACAutoBtnCmd_flg/1 -> AC/26(VINP_HMIACAutoBtnCmd_flg)
  VINP_HMIACBtnCmd_flg/1 -> AC/25(VINP_HMIACBtnCmd_flg)
  EEP_sigSetTempZon2StM/1 -> AC/24(EEP_sigSetTempZon2StM)
  [RemoteAutoReq] -> AC/22(VINP_RemoteAutoReq_flg)
  [ACSubMode] -> AC/23(ACSubMode)
  [TFootRr] -> AC/21(T_Foot_Rr)
  [TFootR] -> AC/20(T_Foot_R)
  VINP_OFFACMODE_enum/1 -> AC/17(OFF_AC_MODE)
  [TFootL] -> AC/19(T_Foot_L)
  [CabinMode] -> AC/18(CabinMode)
  VINP_sigSetTempZon2Req_C/1 -> AC/14(VINP_sigSetTempZon2Req_C)
  VINP_CANMsgValidIVI2_flg/1 -> AC/13(VINP_CANMsgValidIVI2_flg)
  [PwrSta] -> AC/16(PwrSta)
  [FD_Blower_Cmd] -> AC/15(VTHC_FDBlowerCmd_pct)
  VINP_sigSetTempZon1Req_C/1 -> AC/12(VINP_sigSetTempZon1Req_C)
  VINP_sigFrostReq_flg/1 -> AC/11(VINP_sigFrostReq_flg)
  VINP_sigFootReq_flg/1 -> AC/10(VINP_sigFootReq_flg)
  VINP_sigFaceReq_flg/1 -> AC/9(VINP_sigFaceReq_flg)
  VINP_sigRecircReq_flg/1 -> AC/8(VINP_sigRecircReq_flg)
  VINP_sigAirIntenZon1Req_enum/1 -> AC/7(VINP_sigAirIntenZon1Req_enum)
  VINP_FCPFrEvtBtnSyncReq_flg/1 -> AC/4(VINP_FCPFrEvtBtnSyncReq_flg)
  [Tincar] -> AC/6(VINP_Tincar_C)
  VINP_FCPFrEvtBtnAutoReq_flg/1 -> AC/3(VINP_FCPFrEvtBtnAutoReq_flg)
  [Tamb] -> AC/5(VINP_Tamb_C)
  VINP_FCPFrEvtBtnACReq_flg/1 -> AC/2(VINP_FCPFrEvtBtnACReq_flg)
  VINP_FCPFrEvtBtnACMaxReq_flg/1 -> AC/1(VINP_FCPFrEvtBtnACMaxReq_flg)
  AC/132(FDCTHCCREVentYStaSet3) -> VTHC_FDCTHCCREVentYStaSet3_enum/1  "VTHC_FDCTHCCREVentYStaSet3_enum"
  AC/134(FDCTHCCREVentYStaSet5) -> VTHC_FDCTHCCREVentYStaSet5_enum/1  "VTHC_FDCTHCCREVentYStaSet5_enum"
  AC/141(SettempZon1Set7) -> VTHC_SettempZon1Set7_enum/1  "VTHC_SettempZon1Set7_enum"
  AC/136(SettempZon1Set1) -> VTHC_SettempZon1Set1_enum/1  "VTHC_SettempZon1Set1_enum"
  AC/135(FDCTHCCREVentYStaSet7) -> VTHC_FDCTHCCREVentYStaSet7_enum/1  "VTHC_FDCTHCCREVentYStaSet7_enum"
  AC/133(FDCTHCCREVentYStaSet4) -> VTHC_FDCTHCCREVentYStaSet4_enum/1  "VTHC_FDCTHCCREVentYStaSet4_enum"
  AC/140(SettempZon1Set5) -> VTHC_SettempZon1Set5_enum/1  "VTHC_SettempZon1Set5_enum"
  AC/138(SettempZon1Set3) -> VTHC_SettempZon1Set3_enum/1  "VTHC_SettempZon1Set3_enum"
  AC/137(SettempZon1Set2) -> VTHC_SettempZon1Set2_enum/1  "VTHC_SettempZon1Set2_enum"
  AC/139(SettempZon1Set4) -> VTHC_SettempZon1Set4_enum/1  "VTHC_SettempZon1Set4_enum"
  AC/131(FDCTHCCREVentYStaSet2) -> VTHC_FDCTHCCREVentYStaSet2_enum/1  "VTHC_FDCTHCCREVentYStaSet2_enum"
  AC/128(FDCTHCREventYStaSet5) -> VTHC_FDCTHCREVentYStaSet5_enum/1  "VTHC_FDCTHCREVentYStaSet5_enum"
  AC/130(FDCTHCCREVentYStaSet1) -> VTHC_FDCTHCCREVentYStaSet1_enum/1  "VTHC_FDCTHCCREVentYStaSet1_enum"
  AC/127(FDCTHCREventYStaSet4) -> VTHC_FDCTHCREVentYStaSet4_enum/1  "VTHC_FDCTHCREVentYStaSet4_enum"
  AC/129(FDCTHCREventYStaSet7) -> VTHC_FDCTHCREVentYStaSet7_enum/1  "VTHC_FDCTHCREVentYStaSet7_enum"
  AC/126(FDCTHCREventYStaSet3) -> VTHC_FDCTHCREVentYStaSet3_enum/1  "VTHC_FDCTHCREVentYStaSet3_enum"
  AC/125(FDCTHCREventYStaSet2) -> VTHC_FDCTHCREVentYStaSet2_enum/1  "VTHC_FDCTHCREVentYStaSet2_enum"
  AC/124(FDCTHCREventYStaSet1) -> VTHC_FDCTHCREVentYStaSet1_enum/1  "VTHC_FDCTHCREVentYStaSet1_enum"
  AC/123(FDCTHCCLEVentYStaSet7) -> VTHC_FDCTHCCLEVentYStaSet7_enum/1  "VTHC_FDCTHCCLEVentYStaSet7_enum"
  AC/122(FDCTHCCLEVentYStaSet5) -> VTHC_FDCTHCCLEVentYStaSet5_enum/1  "VTHC_FDCTHCCLEVentYStaSet5_enum"
  AC/121(FDCTHCCLEVentYStaSet4) -> VTHC_FDCTHCCLEVentYStaSet4_enum/1  "VTHC_FDCTHCCLEVentYStaSet4_enum"
  AC/120(FDCTHCCLEVentYStaSet3) -> VTHC_FDCTHCCLEVentYStaSet3_enum/1  "VTHC_FDCTHCCLEVentYStaSet3_enum"
  AC/119(FDCTHCCLEVentYStaSet2) -> VTHC_FDCTHCCLEVentYStaSet2_enum/1  "VTHC_FDCTHCCLEVentYStaSet2_enum"
  AC/118(FDCTHCCLEVentYStaSet1) -> VTHC_FDCTHCCLEVentYStaSet1_enum/1  "VTHC_FDCTHCCLEVentYStaSet1_enum"
  AC/117(FDCTHCLEventYStaSet7) -> VTHC_FDCTHCLEVentYStaSet7_enum/1  "VTHC_FDCTHCLEVentYStaSet7_enum"
  AC/116(FDCTHCLEventYStaSet5) -> VTHC_FDCTHCLEVentYStaSet5_enum/1  "VTHC_FDCTHCLEVentYStaSet5_enum"
  AC/115(FDCTHCLEventYStaSet4) -> VTHC_FDCTHCLEVentYStaSet4_enum/1  "VTHC_FDCTHCLEVentYStaSet4_enum"
  AC/114(FDCTHCLEventYStaSet3) -> VTHC_FDCTHCLEVentYStaSet3_enum/1  "VTHC_FDCTHCLEVentYStaSet3_enum"
  AC/113(FDCTHCLEventYStaSet2) -> VTHC_FDCTHCLEVentYStaSet2_enum/1  "VTHC_FDCTHCLEVentYStaSet2_enum"
  AC/112(FDCTHCLEventYStaSet1) -> VTHC_FDCTHCLEVentYStaSet1_enum/1  "VTHC_FDCTHCLEVentYStaSet1_enum"
  AC/110(FDCTHCCREVentZStaSet5) -> VTHC_FDCTHCCREVentZStaSet5_enum/1  "VTHC_FDCTHCCREVentZStaSet5_enum"
  AC/109(FDCTHCCREVentZStaSet4) -> VTHC_FDCTHCCREVentZStaSet4_enum/1  "VTHC_FDCTHCCREVentZStaSet4_enum"
  AC/111(FDCTHCCREVentZStaSet7) -> VTHC_FDCTHCCREVentZStaSet7_enum/1  "VTHC_FDCTHCCREVentZStaSet7_enum"
  AC/108(FDCTHCCREVentZStaSet3) -> VTHC_FDCTHCCREVentZStaSet3_enum/1  "VTHC_FDCTHCCREVentZStaSet3_enum"
  AC/107(FDCTHCCREVentZStaSet2) -> VTHC_FDCTHCCREVentZStaSet2_enum/1  "VTHC_FDCTHCCREVentZStaSet2_enum"
  AC/106(FDCTHCCREVentZStaSet1) -> VTHC_FDCTHCCREVentZStaSet1_enum/1  "VTHC_FDCTHCCREVentZStaSet1_enum"
  AC/101(FDCTHCREventZStaSet2) -> VTHC_FDCTHCREVentZStaSet2_enum/1  "VTHC_FDCTHCREVentZStaSet2_enum"
  AC/105(FDCTHCREventZStaSet7) -> VTHC_FDCTHCREVentZStaSet7_enum/1  "VTHC_FDCTHCREVentZStaSet7_enum"
  AC/102(FDCTHCREventZStaSet3) -> VTHC_FDCTHCREVentZStaSet3_enum/1  "VTHC_FDCTHCREVentZStaSet3_enum"
  AC/100(FDCTHCREventZStaSet1) -> VTHC_FDCTHCREVentZStaSet1_enum/1  "VTHC_FDCTHCREVentZStaSet1_enum"
  AC/103(FDCTHCREventZStaSet4) -> VTHC_FDCTHCREVentZStaSet4_enum/1  "VTHC_FDCTHCREVentZStaSet4_enum"
  AC/104(FDCTHCREventZStaSet5) -> VTHC_FDCTHCREVentZStaSet5_enum/1  "VTHC_FDCTHCREVentZStaSet5_enum"
  AC/99(FDCTHCCLEVentZStaSet7) -> VTHC_FDCTHCCLEVentZStaSet7_enum/1  "VTHC_FDCTHCCLEVentZStaSet7_enum"
  AC/98(FDCTHCCLEVentZStaSet5) -> VTHC_FDCTHCCLEVentZStaSet5_enum/1  "VTHC_FDCTHCCLEVentZStaSet5_enum"
  AC/97(FDCTHCCLEVentZStaSet4) -> VTHC_FDCTHCCLEVentZStaSet4_enum/1  "VTHC_FDCTHCCLEVentZStaSet4_enum"
  AC/96(FDCTHCCLEVentZStaSet3) -> VTHC_FDCTHCCLEVentZStaSet3_enum/1  "VTHC_FDCTHCCLEVentZStaSet3_enum"
  AC/95(FDCTHCCLEVentZStaSet2) -> VTHC_FDCTHCCLEVentZStaSet2_enum/1  "VTHC_FDCTHCCLEVentZStaSet2_enum"
  AC/93(FDCTHCLEventZStaSet7) -> VTHC_FDCTHCLEVentZStaSet7_enum/1  "VTHC_FDCTHCLEVentZStaSet7_enum"
  AC/92(FDCTHCLEventZStaSet5) -> VTHC_FDCTHCLEVentZStaSet5_enum/1  "VTHC_FDCTHCLEVentZStaSet5_enum"
  AC/94(FDCTHCCLEVentZStaSet1) -> VTHC_FDCTHCCLEVentZStaSet1_enum/1  "VTHC_FDCTHCCLEVentZStaSet1_enum"
  AC/91(FDCTHCLEventZStaSet4) -> VTHC_FDCTHCLEVentZStaSet4_enum/1  "VTHC_FDCTHCLEVentZStaSet4_enum"
  AC/90(FDCTHCLEventZStaSet3) -> VTHC_FDCTHCLEVentZStaSet3_enum/1  "VTHC_FDCTHCLEVentZStaSet3_enum"
  AC/89(FDCTHCLEventZStaSet2) -> VTHC_FDCTHCLEVentZStaSet2_enum/1  "VTHC_FDCTHCLEVentZStaSet2_enum"
  AC/87(FDCTHCREventModeStaSet457) -> VTHC_REVentModeStaSet457_enum/1  "VTHC_REVentModeStaSet457_enum"
  AC/88(FDCTHCLEventZStaSet1) -> VTHC_FDCTHCLEVentZStaSet1_enum/1  "VTHC_FDCTHCLEVentZStaSet1_enum"
  AC/86(FDCTHCREventModeStaSet123) -> VTHC_REVentModeStaSet123_enum/1  "VTHC_REVentModeStaSet123_enum"
  AC/85(FDCTHCLEventModeStaSet457) -> VTHC_LEVentModeStaSet457_enum/1  "VTHC_LEVentModeStaSet457_enum"
  AC/84(FDCTHCLEventModeStaSet123) -> VTHC_LEVentModeStaSet123_enum/1  "VTHC_LEVentModeStaSet123_enum"
  AC/83(CRVentENSet) -> VTHC_CRVentENSet_enum/1  "VTHC_CRVentENSet_enum"
  AC/82(RVentENSet) -> VTHC_RVentENSet_enum/1  "VTHC_RVentENSet_enum"
  AC/81(CLVentENSet) -> VTHC_CLVentENSet_enum/1  "VTHC_CLVentENSet_enum"
  AC/80(LVentENSet) -> VTHC_LVentENSet_enum/1  "VTHC_LVentENSet_enum"
  AC/79(FDCFGSAirIntStaSet457) -> VTHC_FDCFGSAirIntStaSet457_enum/1  "VTHC_FDCFGSAirIntStaSet457_enum"
  AC/78(FDCFGSAirIntStaSet123) -> VTHC_FDCFGSAirIntStaSet123_enum/1  "VTHC_FDCFGSAirIntStaSet123_enum"
  AC/77(FDCFGSChStaSet457) -> VTHC_FDCFGSChStaSet457_enum/1  "VTHC_FDCFGSChStaSet457_enum"
  AC/76(FDCFGSChStaSet123) -> VTHC_FDCFGSChStaSet123_enum/1  "VTHC_FDCFGSChStaSet123_enum"
  AC/75(IONSWStaSet) -> VTHC_IONSWStaSet_enum/1  "VTHC_IONSWStaSet_enum"
  AC/74(AirIntenZone3MSet7) -> VTHC_AirIntenZone3MSet7_enum/1  "VTHC_AirIntenZone3MSet7_enum"
  AC/73(AirIntenZone3MSet5) -> VTHC_AirIntenZone3MSet5_enum/1  "VTHC_AirIntenZone3MSet5_enum"
  AC/72(AirIntenZone3MSet4) -> VTHC_AirIntenZone3MSet4_enum/1  "VTHC_AirIntenZone3MSet4_enum"
  AC/71(AirIntenZone3MSet3) -> VTHC_AirIntenZone3MSet3_enum/1  "VTHC_AirIntenZone3MSet3_enum"
  AC/70(AirIntenZone3MSet2) -> VTHC_AirIntenZone3MSet2_enum/1  "VTHC_AirIntenZone3MSet2_enum"
  AC/69(AirIntenZone3MSet1) -> VTHC_AirIntenZone3MSet1_enum/1  "VTHC_AirIntenZone3MSet1_enum"
  AC/68(AirIntenZone1MSet7) -> VTHC_AirIntenZone1MSet7_enum/1  "VTHC_AirIntenZone1MSet7_enum"
  AC/67(AirIntenZone1MSet5) -> VTHC_AirIntenZone1MSet5_enum/1  "VTHC_AirIntenZone1MSet5_enum"
  AC/66(AirIntenZone1MSet4) -> VTHC_AirIntenZone1MSet4_enum/1  "VTHC_AirIntenZone1MSet4_enum"
  AC/65(AirIntenZone1MSet3) -> VTHC_AirIntenZone1MSet3_enum/1  "VTHC_AirIntenZone1MSet3_enum"
  AC/64(AirIntenZone1MSet2) -> VTHC_AirIntenZone1MSet2_enum/1  "VTHC_AirIntenZone1MSet2_enum"
  AC/63(AirIntenZone1MSet1) -> VTHC_AirIntenZone1MSet1_enum/1  "VTHC_AirIntenZone1MSet1_enum"
  AC/62(RecyAutoSet) -> VTHC_RecyAutoSet_enum/1  "VTHC_RecyAutoSet_enum"
  AC/61(sigRecircStSet) -> VTHC_sigRecircStSet_enum/1  "VTHC_sigRecircStSet_enum"
  AC/60(CCUSyncStsSet) -> VTHC_CCUSyncStsSet_enum/1  "VTHC_CCUSyncStsSet_enum"
  AC/59(fdefogSet) -> VTHC_fdefogSet_enum/1  "VTHC_fdefogSet_enum"
  AC/58(FootMSet) -> VTHC_FootMSet_enum/1  "VTHC_FootMSet_enum"
  AC/57(FaceMSet) -> VTHC_FaceMSet_enum/1  "VTHC_FaceMSet_enum"
  THCM_Conctrl/50(VTHC_EWPBUflag3_flg) -> VTHC_EWPBUflag3_flg/1  "VTHC_EWPBUflag3_flg"
  THCM_Conctrl/49(VTHC_EWPBUflag2_flg) -> VTHC_EWPBUflag2_flg/1  "VTHC_EWPBUflag2_flg"
  THCM_Conctrl/48(VTHC_EWPBUflag1_flg) -> VTHC_EWPBUflag1_flg/1  "VTHC_EWPBUflag1_flg"
  VINP_EWP3OverCurrError_enum/1 -> THCM_Conctrl/100(VINP_EWP3OverCurrError_enum)
  VINP_EWP3BlockError_enum/1 -> THCM_Conctrl/99(VINP_EWP3BlockError_enum)
  VINP_EWP2OverCurrError_enum/1 -> THCM_Conctrl/98(VINP_EWP2OverCurrError_enum)
  VINP_EWP2BlockError_enum/1 -> THCM_Conctrl/97(VINP_EWP2BlockError_enum)
  VINP_EWP1OverCurrError_enum/1 -> THCM_Conctrl/96(VINP_EWP1OverCurrError_enum)
  "VINP_EWP1BlockError_enum "/1 -> THCM_Conctrl/95("VINP_EWP1BlockError_enum ")
  THCM_Conctrl/47(VTHC_FDCTHCMPreWPTCHeatSta_enum) -> VTHC_FDCTHCMPreWPTCHeatSta_enum/1
  VINP_IVIWPTCSWSta_flg/1 -> THCM_Conctrl/93(VINP_IVIWPTCSWSta_flg)
  VINP_HVBattSOC_pct/1 -> THCM_Conctrl/92(VINP_HVBattSOCDis_pct)
  [sigWindDirZon1St] -> THCM_Conctrl/94(sigWindDirZon1St)
  Unit Delay14/1 -> [sigWindDirZon1St]
  [VTHC_FDCTHCMAPTCForceOFFSta_flg] -> Unit Delay13/1
  Unit Delay13/1 -> THCM_Conctrl/90(APTCFailDTC)
  APTCFailDTC/1 -> Terminator/1
  THCM_Conctrl/46(VTHC_FDCTHCMAPTCForceOFFSta_flg) -> Data Type Conversion50/1, [VTHC_FDCTHCMAPTCForceOFFSta_flg]
  Data Type Conversion50/1 -> VTHC_FDCTHCMAPTCForceOFFSta_flg/1  "VTHC_FDCTHCMAPTCForceOFFSta_flg"
  AC/40(VTHC_FDCTHCCRVentENSta_flg) -> VTHC_FDCTHCCRVentENSta_flg/1  "VTHC_FDCTHCCRVentENSta_flg"
  AC/39(VTHC_FDCTHCCREVentYSta_enum) -> VTHC_FDCTHCCREVentYSta_enum/1  "VTHC_FDCTHCCREVentYSta_enum"
  AC/38(VTHC_FDCTHCRVentENSta_flg) -> VTHC_FDCTHCRVentENSta_flg/1  "VTHC_FDCTHCRVentENSta_flg"
  AC/37(VTHC_FDCTHCREventYSta_enum) -> VTHC_FDCTHCREVentYSta_enum/1  "VTHC_FDCTHCREVentYSta_enum"
  AC/36(VTHC_FDCTHCCLVentENSta_flg) -> VTHC_FDCTHCCLVentENSta_flg/1  "VTHC_FDCTHCCLVentENSta_flg"
  AC/35(VTHC_FDCTHCCLEVentYSta_enum) -> VTHC_FDCTHCCLEVentYSta_enum/1  "VTHC_FDCTHCCLEVentYSta_enum"
  AC/34(VTHC_FDCTHCLVentENSta_flg) -> VTHC_FDCTHCLVentENSta_flg/1  "VTHC_FDCTHCLVentENSta_flg"
  AC/33(VTHC_FDCTHCLEventYSta_enum) -> VTHC_FDCTHCLEVentYSta_enum/1  "VTHC_FDCTHCLEVentYSta_enum"
  AC/32(VTHC_FDCTHCCREVentZSta_enum) -> VTHC_FDCTHCCREVentZSta_enum/1  "VTHC_FDCTHCCREVentZSta_enum"
  AC/31(VTHC_FDCTHCREventZSta_enum) -> VTHC_FDCTHCREVentZSta_enum/1  "VTHC_FDCTHCREVentZSta_enum"
  AC/30(VTHC_FDCTHCCLEVentZSta_enum) -> VTHC_FDCTHCCLEVentZSta_enum/1  "VTHC_FDCTHCCLEVentZSta_enum"
  AC/29(VTHC_FDCTHCLEventZSta_enum) -> VTHC_FDCTHCLEVentZSta_enum/1  "VTHC_FDCTHCLEVentZSta_enum"
  AC/28(VTHC_FDCTHCREventModeSta_enum) -> VTHC_FDCTHCREVentModeSta_enum/1  "VTHC_FDCTHCREVentModeSta_enum"
  AC/27(VTHC_FDCTHCLEventModeSta_enum) -> VTHC_FDCTHCLEVentModeSta_enum/1  "VTHC_FDCTHCLEVentModeSta_enum"
  [RrAPTCEN] -> Unit Delay6/1
  Unit Delay12/1 -> [RrAPTCEN]
  AC/26(RrAPTCEN) -> Unit Delay12/1
  AC/25(VTHC_FDCTHCAirIntZ3Sta_enum) -> VTHC_FDCTHCAirIntZ3Sta_enum/1
  AC/24(VTHC_sigDfrstSt_flg) -> VTHC_sigDfrstSt_flg/1
  Unit Delay6/1 -> THCM_Conctrl/91(RrAPTCEN)
  VINP_FrntPTCRiActHeatPwr_W/1 -> THCM_Conctrl/89(VINP_FrntPTCRiActHeatPwr_W)
  VINP_FrntPTCLeActHeatPwr_W/1 -> THCM_Conctrl/88(VINP_FrntPTCLeActHeatPwr_W)
  VINP_FrntPTCRearLeActHeatPwr_W/1 -> THCM_Conctrl/87(VINP_FrntPTCRearLeActHeatPwr_W)
  VINP_HVBHVILErr_flg/1 -> THCM_Conctrl/86(VINP_HVBHVILErr_flg)
  VINP_HVBIsoImpedenceP_Mohm/1 -> THCM_Conctrl/85(VINP_HVBIsoImpedenceP_Mohm)
  VINP_HVBIsoImpedenceN_Mohm/1 -> THCM_Conctrl/84(VINP_HVBIsoImpedenceN_Mohm)
  VINP_SmartEcoModeSW_flg/1 -> THCM_Conctrl/83(VINP_SmartEcoModeSW_flg)
  [VINP_COMP_StatorSpd_RPM] -> THCM_Conctrl/31(CompFB)
  Data Type Conversion49/1 -> [VINP_COMP_StatorSpd_RPM]
  Data Type Conversion48/1 -> [EACProtectEnable]
  Unit Delay/1 -> [ACSubMode]
  [RemoteAutoReq] -> THCM_Conctrl/82(RemoteAutoReq)
  VINP_RemoteAutoReq_flg/1 -> [RemoteAutoReq]
  [RemoteACTemp] -> THCM_Conctrl/81(RemoteACTemp)
  VINP_RemoteACTemp_C/1 -> [RemoteACTemp]
  ECOSW/1 -> THCM_Conctrl/80(ECOSW)
  AC/23(VTHC_sigSetTempZon2StM_C) -> VTHC_sigSetTempZon2StM_C/1
  AC/20(RecAutoFlg) -> VTHC_RecAutoFlg_flg/1
  AC/22(fdefog) -> Unit Delay8/1, VTHC_fdefog_flg/1
  AC/21(AirIntenZone1M) -> VTHC_AirIntenZone1M_enum/1
  AC/19(CCUSyncSts) -> VTHC_CCUSyncSts_flg/1
  AC/18(FootM) -> VTHC_FootM_flg/1
  AC/17(FaceM) -> VTHC_FaceM_flg/1
  AC/15(Foot) -> VTHC_Foot_flg/1
  AC/14(Face) -> VTHC_Face_flg/1
  AC/13(ACModeMem) -> VTHC_ACModeMem_enum/1
  SOTXV_Err/1 -> THCM_Conctrl/79(SOTXV_Err)
  PT_Low_T2_Err/1 -> THCM_Conctrl/78(PT_Low_T2_Err)
  PT_Low_P2_Err/1 -> THCM_Conctrl/77(PT_Low_P2_Err)
  PT_Low_T1_Err/1 -> THCM_Conctrl/76(PT_Low_T1_Err)
  PT_Low_P1_Err/1 -> THCM_Conctrl/75(PT_Low_P1_Err)
  Blower_Err/1 -> THCM_Conctrl/74(Blower_Err)
  Comp_Err/1 -> THCM_Conctrl/73(Comp_Err)
  EXV2_Err/1 -> THCM_Conctrl/72(EXV2_Err)
  EXV1_Err/1 -> THCM_Conctrl/71(EXV1_Err)
  SOV3_Err/1 -> THCM_Conctrl/70(SOV3_Err)
  SOV2_Err/1 -> THCM_Conctrl/69(SOV2_Err)
  SOV1_Err/1 -> THCM_Conctrl/68(SOV1_Err)
  PT_High_Tact_Err/1 -> THCM_Conctrl/67(PT_High_Tact_Err)
  PT_High_P_Err/1 -> THCM_Conctrl/66(PT_High_P_Err)
  EWP3_Err/1 -> THCM_Conctrl/65(EWP3_Err)
  AGS_Err/1 -> THCM_Conctrl/64(AGS_Err)
  Fan_Err/1 -> THCM_Conctrl/63(Fan_Err)
  Motor_Out_Temp_Err/1 -> THCM_Conctrl/62(Motor_Out_Temp_Err)
  Motor_In_Temp_Err/1 -> THCM_Conctrl/61(Motor_In_Temp_Err)
  Bat_In_Temp_Err/1 -> THCM_Conctrl/60(Bat_In_Temp_Err)
  Tincar_Err/1 -> THCM_Conctrl/59(Tincar_Err)
  T_Foot_Rr_Err/1 -> THCM_Conctrl/58(T_Foot_Rr_Err)
  T_Face_Rr_Err/1 -> THCM_Conctrl/57(T_Face_Rr_Err)
  T_Foot_R_Err/1 -> THCM_Conctrl/56(T_Foot_R_Err)
  T_Foot_L_Err/1 -> THCM_Conctrl/55(T_Foot_L_Err)
  T_Face_R_Err/1 -> THCM_Conctrl/54(T_Face_R_Err)
  T_Face_L_Err/1 -> THCM_Conctrl/53(T_Face_L_Err)
  Tevap_Err/1 -> THCM_Conctrl/52(Tevap_Err)
  SolarR_Err/1 -> THCM_Conctrl/51(SolarR_Err)
  SolarL_Err/1 -> THCM_Conctrl/50(SolarL_Err)
  Tamb_Err/1 -> THCM_Conctrl/49(Tamb_Err)
  VINP_TFaceRr_C/1 -> THCM_Conctrl/45(T_Face_Rr)
  VINP_TFaceR_C/1 -> THCM_Conctrl/42(T_Face_R)
  [EACProtectEnable] -> THCM_Conctrl/48(EACProtectEnable)
  [TFootRr] -> THCM_Conctrl/46(T_Foot_Rr)
  [PET] -> THCM_Conctrl/47(PET)
  VINP_TFaceL_C/1 -> THCM_Conctrl/41(T_Face_L)
  VINP_RrLLCTemp_C/1 -> THCM_Conctrl/40(Rr_LLCTemp)
  [TFootL] -> THCM_Conctrl/43(T_Foot_L)
  VINP_FrLLCTemp_C/1 -> THCM_Conctrl/39(Fr_LLCTemp)
  [TFootR] -> THCM_Conctrl/44(T_Foot_R)
  VINP_ChrgPlugSta_enum/1 -> THCM_Conctrl/35(ChrgPlugSta)
  [sigSetTempZon2St] -> THCM_Conctrl/38(sigSetTempZon2St)
  VTQD_ShiftGearPosn_enum/1 -> THCM_Conctrl/34(ShiftGearPosn)
  [WaterFillReq] -> THCM_Conctrl/37(WaterFillReq)
  VSCP_AGSCloseSta_flg/1 -> THCM_Conctrl/33(VSCP_AGSCloseSta_flg)
  [DfrstReq] -> THCM_Conctrl/36(DfrstReq)
  VINP_COMP_StatorSpd_RPM/1 -> Data Type Conversion49/1
  VINP_Tevap_C/1 -> THCM_Conctrl/30(Tevap)
  VINP_MotorOutTemp_C/1 -> THCM_Conctrl/26(Motor_Out_Temp)
  VINP_MotorInTemp_C/1 -> THCM_Conctrl/25(Motor_In_Temp)
  [SolarR] -> THCM_Conctrl/29(SolarR)
  [VINP_CompProEN_flg] -> THCM_Conctrl/32(CompProEN)
  [SolarL] -> THCM_Conctrl/28(SolarL)
  [Tincar] -> THCM_Conctrl/27(Tincar)
  VINP_PTHighTact_C/1 -> THCM_Conctrl/21(PT_High_Tact)
  VINP_PTHighP_kPa/1 -> THCM_Conctrl/20(PT_High_P)
  VINP_PTLowT2_C/1 -> THCM_Conctrl/19(PT_ Low_T2)
  [BatInTemp] -> THCM_Conctrl/23(Bat_In_Temp)
  VINP_PTLowT1_C/1 -> THCM_Conctrl/17(PT_ Low_T1)
  [Tamb] -> THCM_Conctrl/22(Tamb)
  [VINP_BatOutTemp_C] -> THCM_Conctrl/24(Bat_Out_Temp)
  VINP_FrMCUTemp_C/1 -> THCM_Conctrl/15(Fr_MCUTemp)
  VINP_FrTMTemp_C/1 -> THCM_Conctrl/14(Fr_TMTemp)
  VINP_RrMCUTemp_C/1 -> THCM_Conctrl/13(Rr_MCUTemp)
  VINP_RrTMTemp_C/1 -> THCM_Conctrl/12(Rr_TMTemp)
  [PTLowP2] -> THCM_Conctrl/18(PT_Low_P2)
  VINP_DCDCTemp_C/1 -> THCM_Conctrl/11(DCDCTemp)
  VINP_OBCTemp_C/1 -> THCM_Conctrl/10(OBCTemp)
  [PTLowP1] -> THCM_Conctrl/16(PT_ Low_P1)
  VINP_HVBMTempMin_C/1 -> THCM_Conctrl/9(HVBMTempMin)
  VINP_HVBMTempMax_C/1 -> THCM_Conctrl/8(HVBMTempMax)
  VINP_VehSpeed_kph/1 -> THCM_Conctrl/7(VehSpeed)
  [sigAirIntenZon1St] -> THCM_Conctrl/6(sigAirIntenZon1St)
  [sigSetTempZon1St] -> THCM_Conctrl/5(sigSetTempZon1St)
  [ACAUTO] -> THCM_Conctrl/4(ACAuto)
  [ACMAX] -> THCM_Conctrl/3(ACMax)
  [AC] -> THCM_Conctrl/2(AC)
  [PwrSta] -> THCM_Conctrl/1(PwrSta)
  Max/1 -> [PTLowP2]
  Max1/1 -> [PTLowP1]
  VINP_EACProtectEnable_enum/1 -> Switch/3
  Constant2/1 -> Switch/1
  Switch/1 -> Data Type Conversion48/1
  [VINP_CompProEN_flg] -> Switch/2
  AC/12(FD_RecyAuto_Cmd) -> VTHC_FDRecyAutoCmd_enum/1
  Unit Delay11/1 -> [CabinMode]
  Data Type Conversion47/1 -> VTHC_FDCompCmd_rpm/1  "VTHC_FDCompCmd_rpm"
  THCM_Conctrl/1(FD_Comp_Cmd) -> Data Type Conversion47/1
  Unit Delay10/1 -> [PET]
  AC/11(PET) -> Unit Delay10/1
  [VINP_BatOutTemp_C] -> Data Type Conversion40/1
  VINP_BatOutTemp_C/1 -> [VINP_BatOutTemp_C]
  Data Type Conversion46/1 -> VTHC_FDSOTXVCmd_flg/1
  Data Type Conversion/1 -> VTHC_FDBlowerCmd_pct/1
  Unit Delay9/1 -> [sigSetTempZon2St]
  Unit Delay7/1 -> [WaterFillReq]
  Unit Delay8/1 -> [DfrstReq]
  AC/16(Frost) -> VTHC_Frost_flg/1
  AC/10(WaterFillReq) -> Unit Delay7/1
  Data Type Conversion45/1 -> VTHC_sigCbnAirT_C/1  "Tincar"
  Data Type Conversion44/1 -> VTHC_sigAmbAirT_C/1  "Tamb"
  Data Type Conversion43/1 -> VTHC_sigCbnSolarRight_W/1  "SolarR"
  Data Type Conversion42/1 -> VTHC_sigClntTHvBattIn_C/1  "BatInTemp"
  Data Type Conversion41/1 -> VTHC_sigCbnSolarLeft_W/1  "SolarL"
  Data Type Conversion40/1 -> VTHC_sigClntTHvBattOut_C/1  "VINP_BatOutTemp_C"
  Data Type Conversion39/1 -> VTHC_APTCP_K/1  "VTHC_APTCP_K"
  Data Type Conversion38/1 -> VTHC_BlowerI_K/1  "VTHC_BlowerI_K"
  Data Type Conversion37/1 -> VTHC_Vbase_pct/1  "VTHC_Vbase_pct"
  Data Type Conversion36/1 -> VTHC_CompU_K/1  "VTHC_CompU_K"
  Data Type Conversion35/1 -> VTHC_CompI_K/1  "VTHC_CompI_K"
  Data Type Conversion34/1 -> VTHC_CompDeltaU_K/1  "VTHC_CompDeltaU_K"
  Data Type Conversion33/1 -> VTHC_Compe_K/1  "VTHC_Compe_K"
  Data Type Conversion32/1 -> VTHC_Blowere_K/1  "VTHC_Blowere_K"
  Data Type Conversion31/1 -> VTHC_BlowerP_K/1  "VTHC_BlowerP_K"
  Data Type Conversion30/1 -> VTHC_BlowerU_K/1  "VTHC_BlowerU_K"
  Data Type Conversion29/1 -> VTHC_CompP_K/1  "VTHC_CompP_K"
  Data Type Conversion28/1 -> VTHC_ACSubMode_enum/1  "ACSubMode"
  Data Type Conversion27/1 -> VTHC_EXV2e_K/1  "VTHC_EXV2e_K"
  Data Type Conversion26/1 -> VTHC_EXV2U_K/1  "VTHC_EXV2U_K"
  Data Type Conversion25/1 -> VTHC_EXV2I_K/1  "VTHC_EXV2I_K"
  Data Type Conversion24/1 -> VTHC_EXV2P_K/1  "VTHC_EXV2P_K"
  Data Type Conversion23/1 -> VTHC_CabinMode_enum/1  "CabinMode"
  Data Type Conversion22/1 -> VTHC_EDriveMode_enum/1  "EDriveMode"
  Data Type Conversion21/1 -> VTHC_BatteryMode_enum/1  "BatteryMode"
  Data Type Conversion20/1 -> VTHC_FDFrWPTCHeatPwrCmd_W/1  "FD_FrWPTCHeatPwr_Cmd"
  Data Type Conversion19/1 -> VTHC_FDTWVCmd_pct/1  "FD_TWV_Cmd"
  Data Type Conversion18/1 -> VTHC_FDFWVCmd_flg/1  "FD_FWV_Cmd"
  Data Type Conversion17/1 -> VTHC_FDEXV2Cmd_step/1  "FD_EXV2_Cmd"
  THCM_Conctrl/38(VTHC_APTCP_K) -> Data Type Conversion39/1
  Data Type Conversion16/1 -> VTHC_APTCI_K/1  "VTHC_APTCI_K"
  Data Type Conversion15/1 -> VTHC_APTCU_K/1  "VTHC_APTCU_K"
  Data Type Conversion14/1 -> VTHC_APTCe_K/1  "VTHC_APTCe_K"
  Data Type Conversion13/1 -> VTHC_EXV1U_K/1  "VTHC_EXV1U_K"
  Data Type Conversion12/1 -> VTHC_EXV1I_K/1  "VTHC_EXV1I_K"
  Data Type Conversion11/1 -> VTHC_EXV1P_K/1  "VTHC_EXV1P_K"
  Data Type Conversion10/1 -> VTHC_FDEXV1Cmd_step/1  "FD_EXV1_Cmd"
  Data Type Conversion9/1 -> VTHC_EXV1e_K/1  "VTHC_EXV1e_K"
  Data Type Conversion7/1 -> VTHC_FDFrRiAPTCHeatPwrCmd_W/1  "FD_FrRiAPTCHeatPwr_Cmd"
  Data Type Conversion8/1 -> VTHC_FDRrAPTCHeatPwrCmd_W/1  "FD_RrAPTCHeatPwr_Cmd"
  Data Type Conversion6/1 -> VTHC_FDFrLeAPTCHeatPwrCmd_W/1  "FD_FrLeAPTCHeatPwr_Cmd"
  Data Type Conversion5/1 -> VTHC_FDEWP3Cmd_enum/1  "FD_EWP3_Cmd"
  Data Type Conversion4/1 -> VTHC_FDEWP2Cmd_enum/1  "FD_EWP2_Cmd"
  Data Type Conversion3/1 -> VTHC_FDEWP1Cmd_enum/1  "FD_EWP1_Cmd"
  Data Type Conversion2/1 -> VTHC_FDAGSCmd_enum/1  "FD_AGS_Cmd"
  Data Type Conversion1/1 -> VTHC_CoolgFanActDuty_pct/1  "CoolgFanActDuty"
  THCM_Conctrl/5(FD_EXV1_Cmd) -> Data Type Conversion10/1
  THCM_Conctrl/45(VTHC_EXV1e_K) -> Data Type Conversion9/1
  THCM_Conctrl/44(VTHC_EXV1U_K) -> Data Type Conversion13/1
  THCM_Conctrl/43(VTHC_EXV1I_K) -> Data Type Conversion12/1
  THCM_Conctrl/42(VTHC_EXV1P_K) -> Data Type Conversion11/1
  THCM_Conctrl/41(VTHC_APTCe_K) -> Data Type Conversion14/1
  THCM_Conctrl/40(VTHC_APTCU_K) -> Data Type Conversion15/1
  THCM_Conctrl/39(VTHC_APTCI_K) -> Data Type Conversion16/1
  THCM_Conctrl/37(VTHC_EXV2e_K) -> Data Type Conversion27/1
  THCM_Conctrl/36(VTHC_EXV2U_K) -> Data Type Conversion26/1
  THCM_Conctrl/35(VTHC_EXV2I_K) -> Data Type Conversion25/1
  THCM_Conctrl/34(VTHC_EXV2P_K) -> Data Type Conversion24/1
  THCM_Conctrl/33(VTHC_BlowerI_K) -> Data Type Conversion38/1
  THCM_Conctrl/32(VTHC_Vbase_pct) -> Data Type Conversion37/1
  THCM_Conctrl/31(VTHC_BlowerU_K) -> Data Type Conversion30/1
  THCM_Conctrl/30(VTHC_BlowerP_K) -> Data Type Conversion31/1
  THCM_Conctrl/29(VTHC_Blowere_K) -> Data Type Conversion32/1
  THCM_Conctrl/28(VTHC_Compe_K) -> Data Type Conversion33/1
  THCM_Conctrl/27(VTHC_CompDeltaU_K) -> Data Type Conversion34/1
  THCM_Conctrl/26(VTHC_CompU_K) -> Data Type Conversion36/1
  THCM_Conctrl/25(VTHC_CompI_K) -> Data Type Conversion35/1
  THCM_Conctrl/24(VTHC_CompP_K) -> Data Type Conversion29/1
  THCM_Conctrl/23(ACSubMode) -> Unit Delay/1, Data Type Conversion28/1
  VINP_CompProEN_flg/1 -> [VINP_CompProEN_flg]
  VINP_TFootRr_C/1 -> [TFootRr]
  VINP_TFootR_C/1 -> [TFootR]
  VINP_PTLowP1_kPa/1 -> Abs1/1
  Abs1/1 -> Max1/1
  Constant1/1 -> Max1/2
  Constant/1 -> Max/2
  Abs/1 -> Max/1
  VINP_PTLowP2_kPa/1 -> Abs/1
  [Tincar] -> Data Type Conversion45/1  "VTHC_sigCbnAirT_C"
  [Tamb] -> Data Type Conversion44/1  "VTHC_sigAmbAirT_C"
  [BatInTemp] -> Data Type Conversion42/1  "VTHC_sigClntTHvBattIn_C"
  [SolarR] -> Data Type Conversion43/1  "VTHC_sigCbnSolarRight_W"
  [SolarL] -> Data Type Conversion41/1  "VTHC_sigCbnSolarLeft_W"
  THCM_Conctrl/22(CabinMode) -> Data Type Conversion23/1, Unit Delay11/1
  THCM_Conctrl/10(FD_FrWPTCHeatPwr_Cmd) -> Data Type Conversion20/1
  Unit Delay4/1 -> [sigAirIntenZon1St]
  VINP_TFootL_C/1 -> [TFootL]
  THCM_Conctrl/12(FD_AGS_Cmd) -> Data Type Conversion2/1
  VINP_SolarL_W/1 -> [SolarL]
  THCM_Conctrl/17(FD_FrRiAPTCHeatPwr_Cmd) -> Data Type Conversion7/1
  Unit Delay1/1 -> [AC]
  VINP_BatInTemp_C/1 -> [BatInTemp]
  THCM_Conctrl/8(FD_FWV_Cmd) -> Data Type Conversion18/1
  VINP_Tamb_C/1 -> [Tamb]
  THCM_Conctrl/6(FD_EXV2_Cmd) -> Data Type Conversion17/1
  THCM_Conctrl/3(FD_SOV2_Cmd) -> VTHC_FDSOV2Cmd_flg/1
  THCM_Conctrl/14(FD_EWP2_Cmd) -> Data Type Conversion4/1
  THCM_Conctrl/7(FD_SOTXV_Cmd) -> Data Type Conversion46/1
  Unit Delay2/1 -> [ACAUTO]
  THCM_Conctrl/2(FD_SOV1_Cmd) -> VTHC_FDSOV1Cmd_flg/1
  THCM_Conctrl/15(FD_EWP3_Cmd) -> Data Type Conversion5/1
  VINP_SolarR_W/1 -> [SolarR]
  THCM_Conctrl/4(FD_SOV3_Cmd) -> VTHC_FDSOV3Cmd_flg/1
  THCM_Conctrl/9(FD_TWV_Cmd) -> Data Type Conversion19/1
  VINP_Tincar_C/1 -> [Tincar]
  THCM_Conctrl/16(FD_FrLeAPTCHeatPwr_Cmd) -> Data Type Conversion6/1
  THCM_Conctrl/20(BatteryMode) -> Data Type Conversion21/1
  THCM_Conctrl/21(EDriveMode) -> Data Type Conversion22/1
  THCM_Conctrl/18(FD_RrAPTCHeatPwr_Cmd) -> Data Type Conversion8/1
  THCM_Conctrl/11(CoolgFanActDuty) -> Data Type Conversion1/1
  THCM_Conctrl/13(FD_EWP1_Cmd) -> Data Type Conversion3/1
  VPMM_PwrSta_enum/1 -> [PwrSta]
  AC/3(VTHC_CCUACMaxLampSts_flg) -> VTHC_CCUACMaxLampSts_flg/1, Unit Delay3/1
  AC/7(VTHC_sigRecircSt_flg) -> VTHC_sigRecircSt_flg/1
  Unit Delay5/1 -> [sigSetTempZon1St]
  THCM_Conctrl/19(FD_Blower_Cmd) -> [FD_Blower_Cmd], Data Type Conversion/1
  AC/8(VTHC_sigSetTempZon1St_C) -> VTHC_sigSetTempZon1St_C/1, Unit Delay5/1
  AC/5(VTHC_sigAirIntenZon1St_enum) -> VTHC_sigAirIntenZon1St_enum/1, Unit Delay4/1
  AC/1(VTHC_CCUACLampSts_flg) -> VTHC_CCUACLampSts_flg/1, Unit Delay1/1
  AC/4(VTHC_CCUSyncLampSts_flg) -> VTHC_CCUSyncLampSts_flg/1
  Unit Delay3/1 -> [ACMAX]
  AC/6(VTHC_sigWindDirZon1St_enum) -> VTHC_sigWindDirZon1St_enum/1, Unit Delay14/1
  AC/2(VTHC_CCUAutoLampSts_flg) -> VTHC_CCUAutoLampSts_flg/1, Unit Delay2/1
  AC/9(VTHC_sigSetTempZon2St_C) -> VTHC_sigSetTempZon2St_C/1, Unit Delay9/1
  VINP_IVIQuickRefreshSta_flg/1 -> AC/150(VINP_IVIQuickRefreshSta_flg)
  THCM_Conctrl/52(sigCbnPTCPwrAct​) -> VTHC_sigCbnPTCPwrAct_W/1  "VTHC_sigCbnPTCPwrAct_W"
